simulink model "q_qube2_swingup"  (R2021a)
settings: Solver=ode1  StartTime=0.0  StopTime=10  FixedStep=Tc  RelTol=1e-3  EnableMultiTasking=on
values from neighbouring files (symbols this model uses):
  actInfo = [-0.05 0 0.05]    [Q-Learning-Deploy.mat]    (also in setup_swingup.m = (-1:1)*tau_max)
  buckets = 8    [Q-Learning-Deploy.mat]    (also in setup_swingup.m)
  episode = 0    [Q-Learning-Deploy.mat]    (also in setup_swingup.m)
  Q_init = [0 0 0 0 0 0 0 0 0 0 0 0 ... (12288 elements, 8x8x8x8x3)]    [Q-Learning-Deploy.mat]    (also in Q_init.mat; setup_swingup.m = results.Q)
  tau_max = 0.05    [Q-Learning-Deploy.mat]
undefined symbols (not defined in the file or in its folder): HIL, qc_get_step_size
libraries: quarc_library x3, dspmathops x1
settings Model: SimulationMode=external  ExtModeTrigDuration=10000  Creator=MLevis  LastModifiedBy=magd4814
settings SolverCC: AlgebraicLoopSolver=TrustRegion  PositivePriorityOrder=on  AutoInsertRateTranBlk=on
settings DebuggingCC: UnderspecifiedInitializationDetection=Classic  MergeDetectMultiDrivingBlocksExec=none  SFMachineParentedDataDiag=warning
settings ModelReferenceCC: PropagateSignalLabelsOutOfModel=off
settings SFSimCC: CustomCodeUndefinedFunction=UseInterfaceOnly
settings RTWCC: Description=QUARC Win64 Target Using Toolchain  SystemTargetFile=quarc_win64.tlc  TemplateMakefile=quarc_default_tmf  Toolchain=QUARC win64 | nmake (64-bit Windows)  BuildConfiguration=Faster Runs
settings STFCustomTargetCC: TargetLangStandard=C99 (ISO)  ConcurrentExecutionCompliant=on  SystemTargetFile=quarc_win64.tlc
settings GRTTargetCC: ParMdlRefBuildCompliant=off  CompOptLevelCompliant=off  CombineOutputUpdateFcns=off  MatFileLogging=off  CPPClassGenCompliant=off  GRTInterface=on  ExtMode=on  ExtModeMexFile=quarc_comm

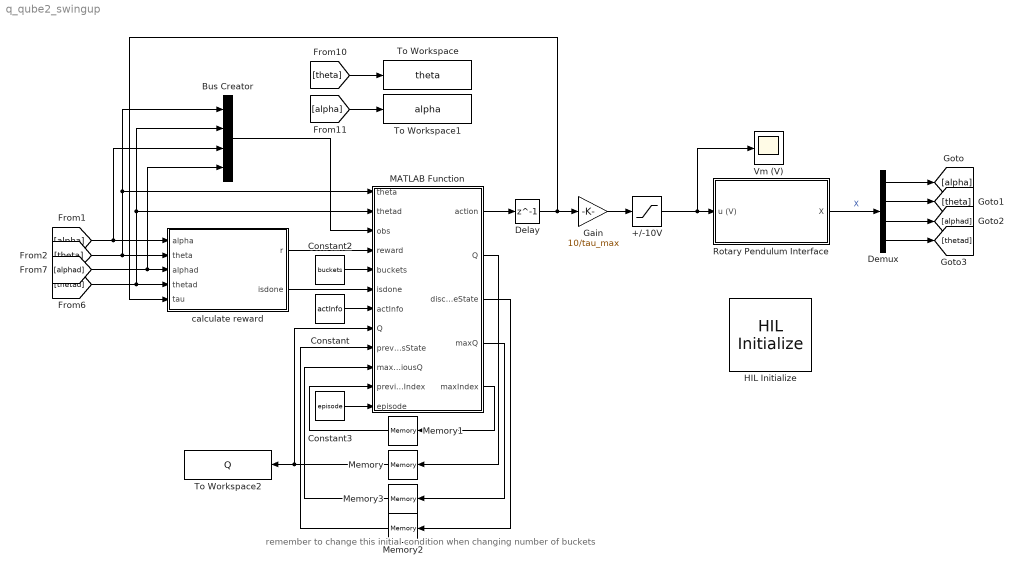
== system q_qube2_swingup ==
  note: remember to change this initial condition when changing number of buckets
  +/-10V : Saturate  UpperLimit=10  LowerLimit=-10
  Bus Creator : BusCreator  Inputs=4
  Constant : Constant  Value=actInfo
  Constant2 : Constant  Value=buckets
  Constant3 : Constant  Value=episode
  Delay : Delay  DelayLength=1
  Demux : Demux
  Gain : Gain  Gain=10/tau_max
  HIL Initialize : quarc_library/Data Acquisition/Generic/Configuration/HIL Initialize  object_name=HIL-1  board_type=qube_servo_usb  board_number=0  board_options=d0=pwm;d1=pwm;led=auto;update_rate=normal;decimation=1  exclusive=off  active=on  hardware_clocks=[0]  clock_modes=[]  initial_clock_frequencies=[]  set_clock_params_at_start=off  set_clock_params_at_switch_in=off  set_clock_frequencies_at_start=off  set_clock_frequencies_at_switch_in=off  analog_input_channels=[]  analog_input_configurations=[]  analog_input_maximums=[]  analog_input_minimums=[]  set_analog_input_params_at_start=off  set_analog_input_params_at_switch_in=off  analog_output_channels=0  analog_output_maximums=10  analog_output_minimums=-10  initial_analog_outputs=[0]  final_analog_outputs=[0]  watchdog_analog_outputs=0  set_analog_output_params_at_start=on  set_analog_output_params_at_switch_in=off  set_analog_outputs_at_start=on  set_analog_outputs_at_switch_in=off  set_analog_outputs_at_terminate=on  set_analog_outputs_at_switch_out=off  set_analog_outputs_on_watchdog=off  digital_input_channels=[]  digital_output_channels=[]  digital_output_configuration=[]  initial_digital_outputs=[]  final_digital_outputs=[]  watchdog_digital_outputs=[]  set_digital_output_params_at_start=off  set_digital_output_params_at_switch_in=off  set_digital_outputs_at_start=off  set_digital_outputs_at_switch_in=off  set_digital_outputs_at_terminate=off  set_digital_outputs_at_switch_out=off  set_digital_outputs_on_watchdog=off  encoder_channels=[0:1]  quadrature=[4]  encoder_filter_frequency=[]  initial_encoder_counts=[0]  set_encoder_params_at_start=on  set_encoder_params_at_switch_in=off  set_encoder_counts_at_start=on  set_encoder_counts_at_switch_in=off  pwm_channels=[]  pwm_modes=[]  pwm_frequency=[]  pwm_configuration=[]  pwm_alignment=[]  pwm_polarity=[]  pwm_leading_deadband=[]  pwm_trailing_deadband=[]  initial_pwm_outputs=[]  final_pwm_outputs=[]  watchdog_pwm_outputs=[]  set_pwm_params_at_start=off  set_pwm_params_at_switch_in=off  set_pwm_outputs_at_start=off  set_pwm_outputs_at_switch_in=off  set_pwm_outputs_at_terminate=off  set_pwm_outputs_at_switch_out=off  set_pwm_outputs_on_watchdog=off  other_output_channels=[]  initial_other_outputs=[]  final_other_outputs=[]  watchdog_other_outputs=[]  set_other_outputs_at_start=off  set_other_outputs_at_switch_in=off  set_other_outputs_at_terminate=off  set_other_outputs_at_switch_out=off  set_other_outputs_on_watchdog=off
  MATLAB Function : MATLAB Function  TreatAsAtomicUnit=on
  Memory : Memory  InitialCondition=Q_init
  Memory1 : Memory  InitialCondition=1
  Memory2 : Memory  InitialCondition=[5 5 5 5]'
  Memory3 : Memory
  Rotary Pendulum Interface : Subsystem
  To Workspace : ToWorkspace  VariableName=theta  SaveFormat=Timeseries  SampleTime=-1
  To Workspace1 : ToWorkspace  VariableName=alpha  SaveFormat=Timeseries  SampleTime=-1
  To Workspace2 : ToWorkspace  VariableName=Q  SampleTime=-1
      settings: MaxDataPoints=1
  Vm (V) : Scope
  calculate reward : Subsystem
  wires:
  Rotary Pendulum Interface/1(X) -> Demux/1  "X"
  Gain/1 -> +/-10V/1
  Demux/1 -> [alpha]
  Demux/2 -> [theta]
  Demux/3 -> [alphad]
  Demux/4 -> [thetad]
  Constant3/1 -> MATLAB Function/12(episode)
  [theta] -> To Workspace/1
  +/-10V/1 -> Vm (V)/1, Rotary Pendulum Interface/1(u (V))
  Constant2/1 -> MATLAB Function/5(buckets)
  [alpha] -> To Workspace1/1
  calculate reward/1(r) -> MATLAB Function/4(reward)
  [alphad] -> Bus Creator/4, calculate reward/3(alphad)
  [thetad] -> MATLAB Function/2(thetad), Bus Creator/2, calculate reward/4(thetad)
  Memory1/1 -> MATLAB Function/11(previousMaxIndex)
  Constant/1 -> MATLAB Function/7(actInfo)
  [theta] -> MATLAB Function/1(theta), Bus Creator/1, calculate reward/2(theta)
  Memory3/1 -> MATLAB Function/10(maxPreviousQ)
  Bus Creator/1 -> MATLAB Function/3(obs)
  Memory/1 -> To Workspace2/1, MATLAB Function/8("Q ")
  Memory2/1 -> MATLAB Function/9(previousState)
  calculate reward/2(isdone) -> MATLAB Function/6(isdone)
  [alpha] -> Bus Creator/3, calculate reward/1(alpha)
  MATLAB Function/1(action) -> Delay/1
  Delay/1 -> calculate reward/5(tau), Gain/1
  MATLAB Function/5(maxIndex) -> Memory1/1
  MATLAB Function/2(Q) -> Memory/1
  MATLAB Function/4(maxQ) -> Memory3/1
  MATLAB Function/3(discreteState) -> Memory2/1

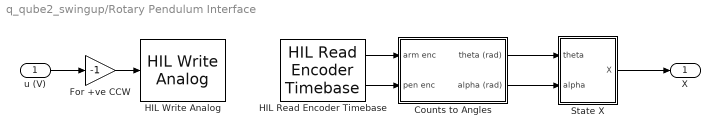
== system q_qube2_swingup/Rotary Pendulum Interface ==
  u (V) : Inport
  Counts to Angles : Subsystem
  For +ve CCW : Gain  Gain=-1
  HIL Read Encoder Timebase : quarc_library/Data Acquisition/Generic/Timebases/HIL Read Encoder Timebase  object_name=HIL-1  clock=0  channels=[0:1]  active=on  vector_output=off  data_type_mode=Inherit via back propagation  data_type=double  overflow_mode=Error on overflow  samples_in_buffer=max(ceil(1/qc_get_step_size), 1)
  HIL Write Analog : quarc_library/Data Acquisition/Generic/Immediate I//O/HIL Write Analog  object_name=HIL-1  channels=0  sample_time=-1  active=on  vector_input=off
  State X : Subsystem
  X : Outport  VectorParamsAs1DForOutWhenUnconnected=off
  wires:
  For +ve CCW/1 -> HIL Write Analog/1
  Counts to Angles/2(alpha (rad)) -> State X/2(alpha)
  Counts to Angles/1(theta (rad)) -> State X/1(theta)
  State X/1(X) -> X/1
  u (V)/1 -> For +ve CCW/1
  HIL Read Encoder Timebase/1 -> Counts to Angles/1(arm enc)
  HIL Read Encoder Timebase/2 -> Counts to Angles/2(pen enc)

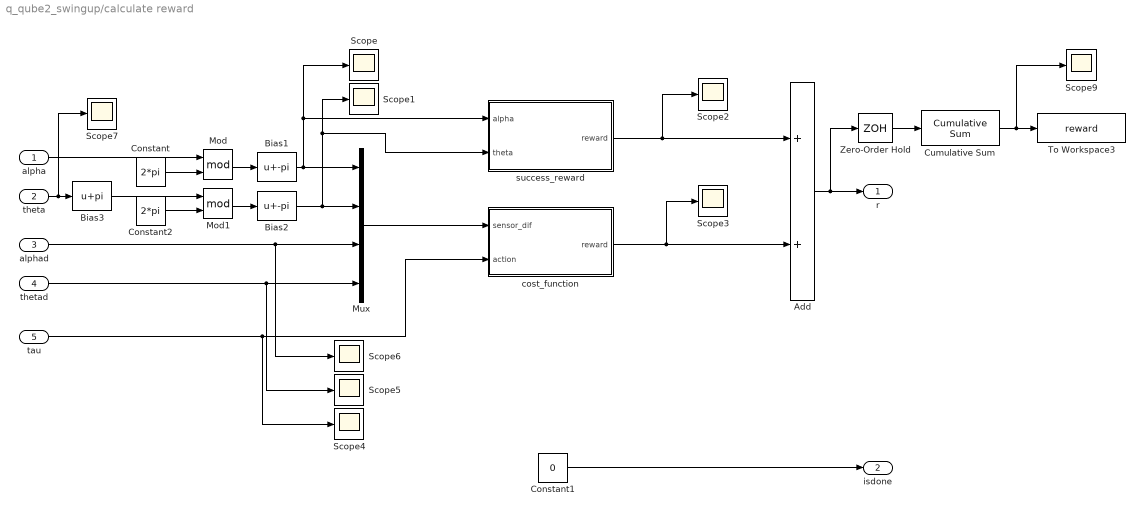
== system q_qube2_swingup/calculate reward ==
  alpha : Inport
  theta : Inport  Port=2
  alphad : Inport  Port=3
  thetad : Inport  Port=4
  tau : Inport  Port=5
  Add : Sum
  Bias1 : Bias  Bias=-pi
  Bias2 : Bias  Bias=-pi
  Bias3 : Bias  Bias=pi
  Constant : Constant  Value=2*pi
  Constant1 : Constant  Value=0
  Constant2 : Constant  Value=2*pi
  Cumulative Sum : dspmathops/Cumulative Sum  dim=Channels (running sum)  InputProcessing=Columns as channels (frame based)  reset_popup=None  roundingMode=Floor  overflowMode=off  outputDataTypeStr=Inherit: Same as accumulator  outputMin=[]  outputMax=[]  outputLastDataTypeStr=Inherit: Same as accumulator
  Mod : Math  Operator=mod  SaturateOnIntegerOverflow=on
  Mod1 : Math  Operator=mod  SaturateOnIntegerOverflow=on
  Mux : Mux
  Scope{,1..7,9} (9 alike) : Scope
  To Workspace3 : ToWorkspace  VariableName=reward  SampleTime=-1
      settings: MaxDataPoints=1
  Zero-Order Hold : ZeroOrderHold  SampleTime=-1
  cost_function : Subsystem
  success_reward : Subsystem
  r : Outport  VectorParamsAs1DForOutWhenUnconnected=off
  isdone : Outport  Port=2  VectorParamsAs1DForOutWhenUnconnected=off
  wires:
  Constant/1 -> Mod/2
  Mod/1 -> Bias1/1
  alpha/1 -> Mod/1
  Bias1/1 -> success_reward/1(alpha), Scope/1, Mux/1
  alphad/1 -> Scope6/1, Mux/3
  tau/1 -> Scope4/1, cost_function/2(action)
  Mux/1 -> cost_function/1(sensor_dif)
  success_reward/1(reward) -> Scope2/1, Add/1
  cost_function/1(reward) -> Scope3/1, Add/2
  Add/1 -> Zero-Order Hold/1, r/1
  Constant1/1 -> isdone/1
  Constant2/1 -> Mod1/2
  theta/1 -> Scope7/1, Bias3/1
  Mod1/1 -> Bias2/1
  Bias2/1 -> Scope1/1, success_reward/2(theta), Mux/2
  Bias3/1 -> Mod1/1
  thetad/1 -> Scope5/1, Mux/4
  Cumulative Sum/1 -> To Workspace3/1, Scope9/1
  Zero-Order Hold/1 -> Cumulative Sum/1

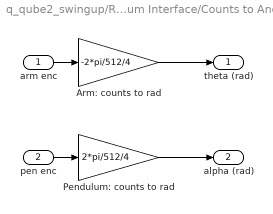
== system q_qube2_swingup/Rotary Pendulum Interface/Counts to Angles ==
  arm enc : Inport
  pen enc : Inport  Port=2
  Arm: counts to rad : Gain  Gain=-2*pi/512/4
  Pendulum: counts to rad : Gain  Gain=2*pi/512/4
  theta (rad) : Outport  VectorParamsAs1DForOutWhenUnconnected=off
  alpha (rad) : Outport  Port=2  VectorParamsAs1DForOutWhenUnconnected=off
  wires:
  pen enc/1 -> Pendulum: counts to rad/1
  arm enc/1 -> Arm: counts to rad/1
  Arm: counts to rad/1 -> theta (rad)/1
  Pendulum: counts to rad/1 -> alpha (rad)/1

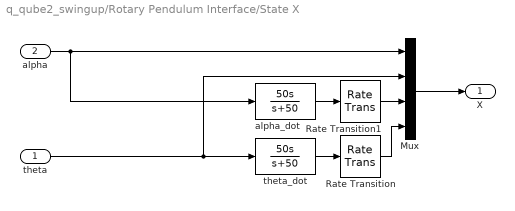
== system q_qube2_swingup/Rotary Pendulum Interface/State X ==
  theta : Inport
  alpha : Inport  Port=2
  Mux : Mux
  Rate Transition : RateTransition
  Rate Transition1 : RateTransition
  alpha_dot : TransferFcn  Numerator=[50 0]  Denominator=[1 50]
  theta_dot : TransferFcn  Numerator=[50 0]  Denominator=[1 50]
  X : Outport  VectorParamsAs1DForOutWhenUnconnected=off
  wires:
  Mux/1 -> X/1
  theta/1 -> Mux/2, theta_dot/1
  alpha/1 -> Mux/1, alpha_dot/1
  theta_dot/1 -> Rate Transition/1
  Rate Transition/1 -> Mux/4
  alpha_dot/1 -> Rate Transition1/1
  Rate Transition1/1 -> Mux/3

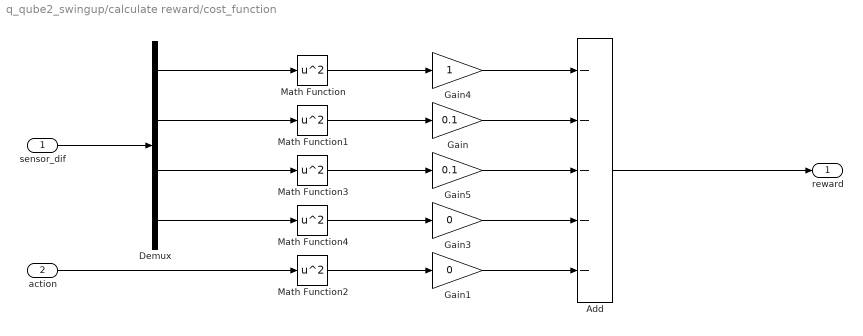
== system q_qube2_swingup/calculate reward/cost_function ==
  sensor_dif : Inport
  action : Inport  Port=2
  Add : Sum  Inputs=-----
  Demux : Demux
  Gain : Gain  Gain=0.1
  Gain1 : Gain  Gain=0
  Gain3 : Gain  Gain=0
  Gain4 : Gain
  Gain5 : Gain  Gain=0.1
  Math Function{,1..4} (5 alike) : Math  Operator=square  SaturateOnIntegerOverflow=on
  reward : Outport
  wires:
  Math Function4/1 -> Gain3/1
  Gain3/1 -> Add/4
  Gain1/1 -> Add/5
  Add/1 -> reward/1
  sensor_dif/1 -> Demux/1
  Demux/4 -> Math Function4/1
  Demux/3 -> Math Function3/1
  Demux/2 -> Math Function1/1
  Math Function1/1 -> Gain/1
  Math Function3/1 -> Gain5/1
  action/1 -> Math Function2/1
  Demux/1 -> Math Function/1
  Math Function2/1 -> Gain1/1
  Gain4/1 -> Add/1
  Gain5/1 -> Add/3
  Gain/1 -> Add/2
  Math Function/1 -> Gain4/1

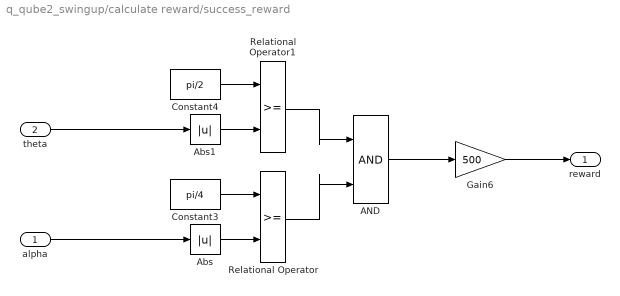
== system q_qube2_swingup/calculate reward/success_reward ==
  alpha : Inport
  theta : Inport  Port=2
  AND : Logic  IconShape=distinctive  AllPortsSameDT=off  OutDataTypeStr=boolean
  Abs : Abs
  Abs1 : Abs
  Constant3 : Constant  Value=pi/4
  Constant4 : Constant  Value=pi/2
  Gain6 : Gain  Gain=500
  Relational Operator : RelationalOperator  OutDataTypeStr=boolean  RndMeth=Simplest
  Relational Operator1 : RelationalOperator  OutDataTypeStr=boolean  RndMeth=Simplest
  reward : Outport
  wires:
  Gain6/1 -> reward/1
  Constant3/1 -> Relational Operator/1
  Abs/1 -> Relational Operator/2
  AND/1 -> Gain6/1
  Relational Operator/1 -> AND/2
  Abs1/1 -> Relational Operator1/2
  Constant4/1 -> Relational Operator1/1
  Relational Operator1/1 -> AND/1
  alpha/1 -> Abs/1
  theta/1 -> Abs1/1

== matlab function q_qube2_swingup/MATLAB Function ==
  settings: updateMethod=DISCRETE
  data: theta input; thetad input; obs input; action output; Q output; reward input; buckets input; isdone input; actInfo input; Q input; previousState input; discreteState output; maxQ output; maxPreviousQ input; previousMaxIndex input; maxIndex output; episode input
function [action,Q,discreteState,maxQ,maxIndex] = fcn(theta,thetad,obs,reward,buckets,isdone,actInfo,Q,previousState,maxPreviousQ,previousMaxIndex,episode)

learningRate = 0;
epsilon = 0;
epsilon_decay = 0;
epsilon_min = 0;
discountFactor = 0.99;

current_epsilon = max(epsilon-epsilon_decay*(episode-1), epsilon_min);

obsHigh = [pi 50 pi 50]';
obsLow = [-pi -50 pi -50]';
 
bucketSize = (obsHigh-obsLow)/buckets;
 
discreteState = floor((obs - obsLow)./bucketSize)+1;
discreteState = min(discreteState,buckets);
discreteState = max(discreteState,1);
 
previousState = min(previousState,buckets);
previousState = max(previousState,1);
 
if theta > 0.65*pi && thetad > -5
    maxIndex = 1;
    action = actInfo(1);
    maxQ = max(Q(discreteState(1),discreteState(2),discreteState(3),discreteState(4),maxIndex));
elseif theta < -0.65*pi && thetad < 5
    maxIndex = 3;
    action = actInfo(3);
    maxQ = max(Q(discreteState(1),discreteState(2),discreteState(3),discreteState(4),maxIndex));
elseif rand()>current_epsilon
    [maxQ,maxIndex] = max(Q(discreteState(1),discreteState(2),discreteState(3),discreteState(4),:));
    action = (maxIndex-2)*actInfo(3);
else
    maxIndex = randi(length(actInfo));
    action = (maxIndex-2)*actInfo(3);
    maxQ = max(Q(discreteState(1),discreteState(2),discreteState(3),discreteState(4),maxIndex));
end

newQ = (1-learningRate)*maxPreviousQ + learningRate*(reward+discountFactor*maxQ);

Q(previousState(1),previousState(2),previousState(3),previousState(4),previousMaxIndex) = newQ;

action = (maxIndex-2)*actInfo(3);
